simulink model "Lewitacja_new"  (R2015a)
settings: Solver=ode5  SolverMode=SingleTasking  StartTime=0.0  StopTime=1000  FixedStep=0.001  RelTol=1e-3  AbsTol=1e-6
PostLoadFcn:
  | load ML_Sensor
values from neighbouring files (symbols this model uses):
  g = model.g    [Levitation.m]
  ki = 2.8964    [Levitation.m]
  m = model.m    [Levitation.m]
  x0 = 0.02    [Levitation.m]
undefined symbols (not defined in the file or in its folder): VIchar
undefined symbols (not defined in the file): Par_Fem, RTDAC4PCIBaseAddress, uc
settings Model: SimulationMode=external  ExtModeEnableFloating=off  ExtModeTrigDuration=40000  ExtModeTrigDirection=either  ExtModeArchiveFileName=exp01.mat  ExtModeArchiveDirName=h:\temp  ExtModeWriteAllDataToWs=on  Creator=Adam Pilat  LastModifiedBy=Student
settings DataIOCC: ExternalInput=[]  InitialState=[]  LimitDataPoints=off  MaxDataPoints=5000  SignalLoggingSaveFormat=ModelDataLogs  SaveOutput=off  SaveTime=off  SignalLoggingName=sigsOut
settings OptimizationCC: BooleanDataType=off  ExpressionDepthLimit=2147483647  InitFltsAndDblsToZero=on
settings DebuggingCC: SaveWithParameterizedLinksMsg=none  UnderspecifiedInitializationDetection=Classic  MergeDetectMultiDrivingBlocksExec=none  SignalResolutionControl=TryResolveAllWithWarning  MultiTaskDSMMsg=warning  MultiTaskCondExecSysMsg=none  IntegerOverflowMsg=none  FcnCallInpInsideContextMsg=UseLocalSettings  StateNameClashWarn=warning  IntegerSaturationMsg=none
settings HardwareCC: ProdBitPerLong=64  ProdBitPerPointer=64  ProdIntDivRoundTo=Zero  ProdEndianess=LittleEndian  ProdWordSize=64  ProdHWDeviceType=Intel->x86-64  TargetBitPerLong=64  TargetBitPerPointer=64  TargetIntDivRoundTo=Zero  TargetEndianess=LittleEndian  TargetWordSize=64  TargetHWDeviceType=Intel->x86-64
settings RTWCC: SystemTargetFile=rtwin.tlc  TemplateMakefile=RTDAC_win.tmf  Description=Real-Time Windows Target
settings RTWinTargetCC: TargetFcnLib=ansi_tfl_tmw.mat  TargetPreCompLibLocation=C:\Program Files\MATLAB\R2015aSP1\toolbox\sldrt\lib\win64  ModelReferenceCompliant=off  CompOptLevelCompliant=off

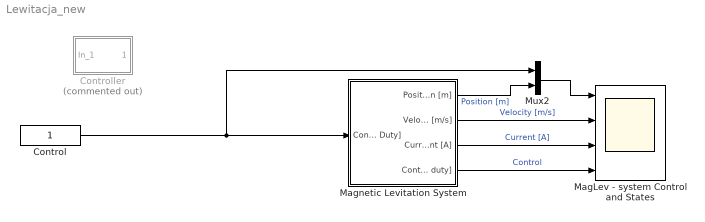
== system Lewitacja_new ==
  Control : Constant
  Controller : Subsystem  Commented=on  mask(PID(2) Controller){P=42, I=16, D=2.1, T0=0.001}
      mask prompts: P "Proportional:"; I "Integral:"; D "Derivative:"; T0 "Sample Time:"
      mask help:
      | Enter Proportional(P), Integral(I), and Derivative(D) and divisor (N) terms.
      | P+I/s+Ds/(1/Ns+1)
      mask Help: This block implements a PID controller where parameters are entered for the Proportional, Integral and Derivative and divisor terms. Unmask this block to see how it works. The derivative term is implemented using an s/(s/N +1)  transfer function block. Making N large can create a "stiff" system.
      mask Display: disp('PID')
  MagLev - system Control and States : Scope  NumInputPorts=4
      settings: TimeRange=10  YMin=2.77556e-17~-0.8~0~0.95  YMax=1~0.7~3~1.05  SaveName=MLExpData  MaxDataPoints=10000
  Magnetic Levitation System : Subsystem  mask(Magnetic Levitation 1 - System){BA=RTDAC4PCIBaseAddress, T0=0.001}
      mask prompts: BA "Base Address (dec):"; T0 "Sampling period [s]:"
      mask help:
      | MagLev1 - System connection for the real-time operating mode
      | (c) InTeCo 2005
      mask Display: image(imread('MagLev1.tif'))
  Mux2 : Mux  Inputs=2
  wires:
  Magnetic Levitation System/1(Position [m]) -> Mux2/2  "Position [m]"
  Magnetic Levitation System/2(Velocity [m/s]) -> MagLev - system Control and States/2  "Velocity [m/s]"
  Magnetic Levitation System/3(Current [A]) -> MagLev - system Control and States/3  "Current [A]"
  Magnetic Levitation System/4(Control [PWM duty]) -> MagLev - system Control and States/4  "Control"
  Mux2/1 -> MagLev - system Control and States/1
  Control/1 -> Mux2/1, Magnetic Levitation System/1(Control [PWM Duty])

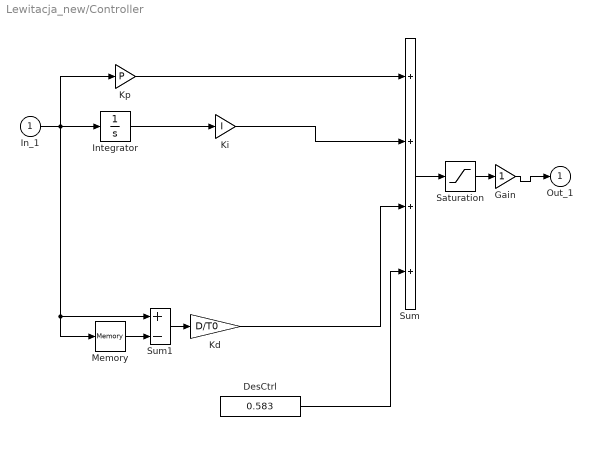
== system Lewitacja_new/Controller ==
  In_1 : Inport
  DesCtrl : Constant  Value=0.583
  Gain : Gain  SaturateOnIntegerOverflow=on  OutDataTypeStr=Inherit: Same as input  ParamDataTypeStr=Inherit: Same as input
  Integrator : Integrator  InitialCondition=0*4e-5  LimitOutput=on  UpperSaturationLimit=1  LowerSaturationLimit=-1
  Kd : Gain  Gain=D/T0  SaturateOnIntegerOverflow=on  OutDataTypeStr=Inherit: Same as input  ParamDataTypeStr=Inherit: Same as input
  Ki : Gain  Gain=I  SaturateOnIntegerOverflow=on  OutDataTypeStr=Inherit: Same as input  ParamDataTypeStr=Inherit: Same as input
  Kp : Gain  Gain=P  SaturateOnIntegerOverflow=on  OutDataTypeStr=Inherit: Same as input  ParamDataTypeStr=Inherit: Same as input
  Memory : Memory
  Saturation : Saturate  UpperLimit=1  LowerLimit=0
  Sum : Sum  Inputs=++++  SaturateOnIntegerOverflow=on  InputSameDT=on  OutDataTypeStr=Inherit: Same as first input
  Sum1 : Sum  Inputs=+-  SaturateOnIntegerOverflow=on  InputSameDT=on  OutDataTypeStr=Inherit: Same as first input
  Out_1 : Outport  InitialOutput=0
  wires:
  Ki/1 -> Sum/2
  Integrator/1 -> Ki/1
  Sum/1 -> Saturation/1
  In_1/1 -> Kp/1, Memory/1, Sum1/1, Integrator/1
  Memory/1 -> Sum1/2
  Sum1/1 -> Kd/1
  DesCtrl/1 -> Sum/4
  Saturation/1 -> Gain/1
  Kp/1 -> Sum/1
  Kd/1 -> Sum/3
  Gain/1 -> Out_1/1

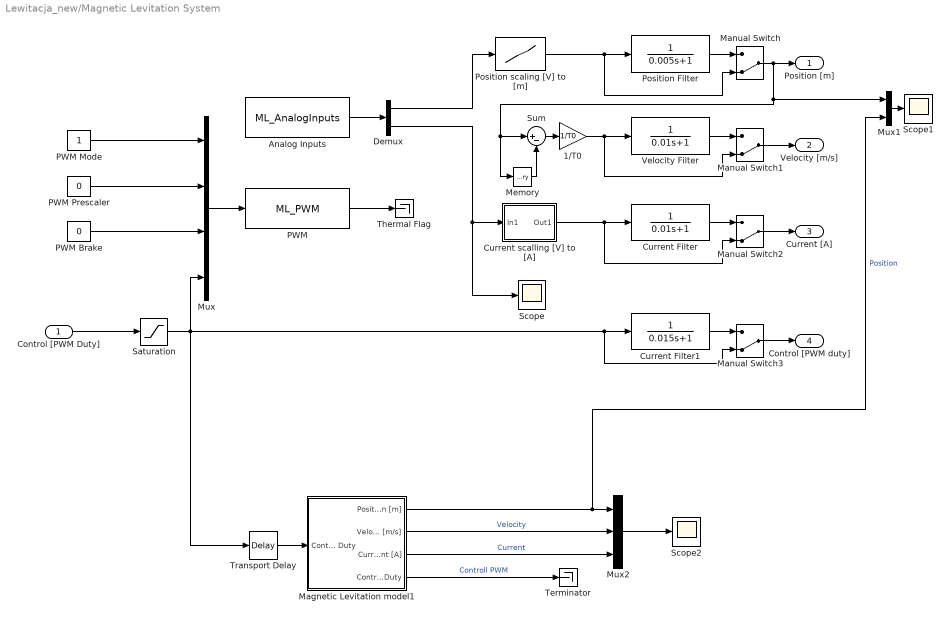
== system Lewitacja_new/Magnetic Levitation System ==
  Control [PWM Duty] : Inport
  1/T0 : Gain  Gain=1/T0  SaturateOnIntegerOverflow=on  OutDataTypeStr=Inherit: Same as input  ParamDataTypeStr=Inherit: Same as input
  Analog Inputs : S-Function  FunctionName=ML_AnalogInputs  Parameters=BA, [4 2], [1 1], T0
  Current Filter : TransferFcn  Denominator=[0.01 1]
  Current Filter1 : TransferFcn  Denominator=[0.015 1]
  Current scalling [V] to [A] : Subsystem
      mask Display: plot([0    0.5000    1.0000    1.5000    2.0000    2.5000], [-0.0317    0.4951    1.0302    1.5738    2.1258    2.6863]);
  Demux : Demux  Outputs=2
  Magnetic Levitation model1 : Subsystem  mask(Magnetic levitation - model){x0=[x0 0 0.3950], m=m, g=g, Par_Fem=Par_Fem, Par_ActStat=[ki, uc], Par_ActDyn=[1.4142e-4, 4.5626e-3], Cnstr=[0, 1, 0.03884, 2.38]}
      mask prompts: x0 "Initial state (position [m], velocity [m/s], current [A]):"; m "Ball mass [kg]"; g "Gravity constant [m/s2]"; Par_Fem "EM Forceparametrs (FemP1 [H], FemP2 [m]):"; Par_ActStat "Actuator parameters (ki [A], ci[A]):"; Par_ActDyn "Actuator parameters fi (fiP1 [m*s], fiP2 [m]):"; Cnstr "Constraints (umin, umax, x3min, x3max):"
      mask help:
      | Nonlinear model of the Magnetic Levitation
      | INTECO (c)
      mask init:
      | ki = Par_ActStat(1);
      | ci = Par_ActStat(2);
      | P1i = Par_ActDyn(1);
      | P2i = Par_ActDyn(2);
      | umin = Cnstr(1);
      | umax = Cnstr(2);
      | x3min = Cnstr(3);
      | x3max = Cnstr(4);
      mask Display:
      | plot(0,0,100,100,[15,5,5,18,82,95,95,85,85,95],[5,5,95,95,95,95,5,5,15,15], [5,15,15,15,25,75,85,85],[15, 15, 5,85,85,85,85,5 ], [50,44,44,38,38,35,35,65,65,62,62,56,56,50],[70,70,81,81,70,70,84,84,70,70,81,81,70,70], [50.00, 50.80, 51.59, 52.36, 53.12, 53.84, 54.52, 55.15, 55.74, 56.27, 56.73, 57.13, 57.46, 57.71, 57.88, 57.98, 58.00, 57.93, 57.79, 57.57, 57.27, 56.91, 56.47, 55.97, 55.40, 54.79, 54.12, 53.42, 52.68, 51.91, 51.13, 50.33, 49.53, 48.74, 47.96, 47.19, 46.46, 45.76, 45.11, 44.50, 43.95, 43.45, 43.03, 42.67, 42.39, 42.18, 42.05, 42.00, 42.03, 42.14, 42.33, 42.59, 42.93, 43.34, 43.82, 44.36, 44.95, 45.59, 46.28, 47.01, 47.76, 48.54, 49.34, ], [58.00, 57.96, 57.84, 57.64, 57.37, 57.02, 56.60, 56.12, 55.57, 54.97, 54.32, 53.63, 52.90, 52.14, 51.36, 50.57, 49.77, 48.97, 48.18, 47.41, 46.67, 45.96, 45.29, 44.67, 44.10, 43.59, 43.14, 42.77, 42.46, 42.23, 42.08, 42.01, 42.01, 42.10, 42.27, 42.51, 42.83, 43.22, 43.67, 44.19, 44.77, 45.40, 46.08, 46.79, 47.54, 48.31, 49.10, 49.90, 50.70, 51.49, 52.27, 53.02, 53.75, 54.43, 55.08, 55.67, 56.20, 56.68, 57.08, 57.42, 57.68, 57.87, 57.97, ],  [15,15,15,85,85,15],[22,28,28,28,22,22])
      | fprintf('\n\n\n\n\nMagLev');
  Manual Switch{,1..3} (4 alike) : ManualSwitch  CurrentSetting=0
  Memory : Memory
  Mux : Mux
  Mux1 : Mux  Inputs=2
  Mux2 : Mux  Inputs=3
  PWM : S-Function  FunctionName=ML_PWM  Parameters=BA, T0
  PWM Brake : Constant  Value=0
  PWM Mode : Constant
  PWM Prescaler : Constant  Value=0
  Position Filter : TransferFcn  Denominator=[0.005 1]
  Position scaling [V] to [m] : Lookup  InputValues=sensor.V(end:-1:1)  Table=sensor.d(end:-1:1)  SaturateOnIntegerOverflow=on
  Saturation : Saturate  UpperLimit=1  LowerLimit=0
  Scope : Scope
      settings: TimeRange=10  YMin=0.77  YMax=0.93
  Scope1 : Scope
      settings: TimeRange=10  YMin=0.005  YMax=0.02
  Scope2 : Scope
      settings: SaveName=ScopeData2
  Sum : Sum  Inputs=|+-  SaturateOnIntegerOverflow=on  InputSameDT=on  OutDataTypeStr=Inherit: Same as first input
  Terminator : Terminator
  Thermal Flag : Terminator
  Transport Delay : TransportDelay  DelayTime=0.01
  Velocity Filter : TransferFcn  Denominator=[0.01 1]
  Position [m] : Outport
  Velocity [m/s] : Outport  Port=2
  Current [A] : Outport  Port=3
  Control [PWM duty] : Outport  Port=4
  wires:
  Current Filter/1 -> Manual Switch2/1
  Velocity Filter/1 -> Manual Switch1/1
  Manual Switch/1 -> Position [m]/1, Mux1/1, Memory/1, Sum/1
  Position Filter/1 -> Manual Switch/1
  Position scaling [V] to [m]/1 -> Manual Switch/2, Position Filter/1
  Demux/1 -> Position scaling [V] to [m]/1
  Demux/2 -> Scope/1, Current scalling [V] to [A]/1(In1)
  Current scalling [V] to [A]/1(Out1) -> Manual Switch2/2, Current Filter/1
  1/T0/1 -> Manual Switch1/2, Velocity Filter/1
  Sum/1 -> 1/T0/1
  Memory/1 -> Sum/2
  Analog Inputs/1 -> Demux/1
  Mux/1 -> PWM/1
  PWM Prescaler/1 -> Mux/2
  PWM Mode/1 -> Mux/1
  PWM/1 -> Thermal Flag/1
  Manual Switch2/1 -> Current [A]/1
  PWM Brake/1 -> Mux/3
  Manual Switch1/1 -> Velocity [m/s]/1
  Control [PWM Duty]/1 -> Saturation/1
  Current Filter1/1 -> Manual Switch3/1
  Manual Switch3/1 -> Control [PWM duty]/1
  Mux1/1 -> Scope1/1
  Magnetic Levitation model1/1(Position [m]) -> Mux1/2, Mux2/1  "Position"
  Magnetic Levitation model1/2(Velocity [m/s]) -> Mux2/2  "Velocity"
  Magnetic Levitation model1/3(Current [A]) -> Mux2/3  "Current"
  Magnetic Levitation model1/4(Control PWMDuty) -> Terminator/1  "Controll PWM"
  Mux2/1 -> Scope2/1
  Transport Delay/1 -> Magnetic Levitation model1/1(Control - PWM Duty)
  Saturation/1 -> Transport Delay/1, Current Filter1/1, Manual Switch3/2, Mux/4

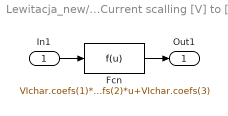
== system Lewitacja_new/Magnetic Levitation System/Current scalling [V] to [A] ==
  In1 : Inport
  Fcn : Fcn  Expr=VIchar.coefs(1)*u^2+VIchar.coefs(2)*u+VIchar.coefs(3)
  Out1 : Outport
  wires:
  In1/1 -> Fcn/1
  Fcn/1 -> Out1/1

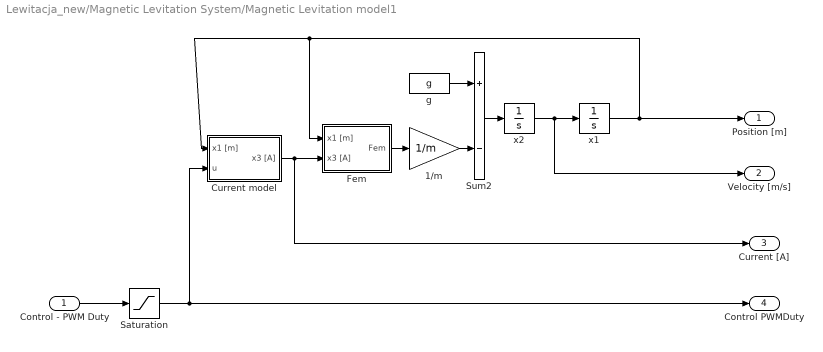
== system Lewitacja_new/Magnetic Levitation System/Magnetic Levitation model1 ==
  Control - PWM Duty : Inport
  1/m : Gain  Gain=1/m  SaturateOnIntegerOverflow=on  OutDataTypeStr=Inherit: Same as input  ParamDataTypeStr=Inherit: Same as input
  Current model : Subsystem
  Fem : Subsystem  mask{FemP1=Par_Fem(1), FemP2=Par_Fem(2)}
  Saturation : Saturate  UpperLimit=umax  LowerLimit=umin
  Sum2 : Sum  Inputs=+-  SaturateOnIntegerOverflow=on  InputSameDT=on  OutDataTypeStr=Inherit: Same as first input
  g : Constant  Value=g
  x1 : Integrator  InitialCondition=x0(1)  LimitOutput=on  UpperSaturationLimit=0.02  LowerSaturationLimit=0.0001
  x2 : Integrator  InitialCondition=x0(2)  UpperSaturationLimit=10  LowerSaturationLimit=-10
  Position [m] : Outport  InitialOutput=0
  Velocity [m/s] : Outport  Port=2  InitialOutput=0
  Current [A] : Outport  Port=3  InitialOutput=0
  Control PWMDuty : Outport  Port=4  InitialOutput=0
  wires:
  Current model/1(x3 [A]) -> Current [A]/1, Fem/2(x3 [A])
  x1/1 -> Position [m]/1, Fem/1(x1 [m]), Current model/1(x1 [m])
  1/m/1 -> Sum2/2
  Fem/1(Fem) -> 1/m/1
  Sum2/1 -> x2/1
  g/1 -> Sum2/1
  x2/1 -> Velocity [m/s]/1, x1/1
  Saturation/1 -> Current model/2(u), Control PWMDuty/1
  Control - PWM Duty/1 -> Saturation/1

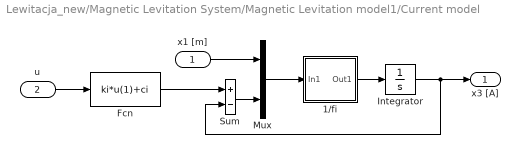
== system Lewitacja_new/Magnetic Levitation System/Magnetic Levitation model1/Current model ==
  x1 [m] : Inport
  u : Inport  Port=2
  1/fi : Subsystem  mask(Current function fi){P1=P1i, P2=P2i}
      mask prompts: P1 "fiP1 [H]:"; P2 "fiP2 [m]:"
      mask Display: plot([0    0.0010    0.0020    0.0030    0.0040    0.0050    0.0060    0.0070   0.0080    0.0090    0.0100    0.0110    0.0120    0.0130    0.0140    0.0150], 1./[0.0292    0.0284    0.0277    0.0271    0.0266    0.0262    0.0258    0.0255    0.0252    0.0250    0.0248    0.0246    0.0245    0.0243    0.0242    0.0241]);
  Fcn : Fcn  Expr=ki*u(1)+ci
  Integrator : Integrator  InitialCondition=x0(3)  LimitOutput=on  UpperSaturationLimit=x3max  LowerSaturationLimit=x3min
  Mux : Mux  Inputs=2
  Sum : Sum  Inputs=+-  SaturateOnIntegerOverflow=on  InputSameDT=on  OutDataTypeStr=Inherit: Same as first input
  x3 [A] : Outport
  wires:
  x1 [m]/1 -> Mux/1
  Mux/1 -> 1/fi/1(In1)
  Sum/1 -> Mux/2
  Fcn/1 -> Sum/1
  Integrator/1 -> Sum/2, x3 [A]/1
  1/fi/1(Out1) -> Integrator/1
  u/1 -> Fcn/1

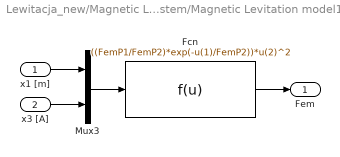
== system Lewitacja_new/Magnetic Levitation System/Magnetic Levitation model1/Fem ==
  x1 [m] : Inport
  x3 [A] : Inport  Port=2
  Fcn : Fcn  Expr=((FemP1/FemP2)*exp(-u(1)/FemP2))*u(2)^2
  Mux3 : Mux  Inputs=2
  Fem : Outport
  wires:
  Mux3/1 -> Fcn/1
  x3 [A]/1 -> Mux3/2
  x1 [m]/1 -> Mux3/1
  Fcn/1 -> Fem/1

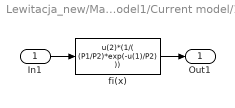
== system Lewitacja_new/Magnetic Levitation System/Magnetic Levitation model1/Current model/1//fi ==
  In1 : Inport
  fi(x) : Fcn  Expr=u(2)*(1/( (P1/P2)*exp(-u(1)/P2) ))
  Out1 : Outport
  wires:
  In1/1 -> fi(x)/1
  fi(x)/1 -> Out1/1
